simulink model "swing_equation_model_without_damping"  (R2014a)
settings: Solver=ode23t  StartTime=0.0  StopTime=3  RelTol=1e-3
settings Model: Creator=Divya M  LastModifiedBy=Divya M

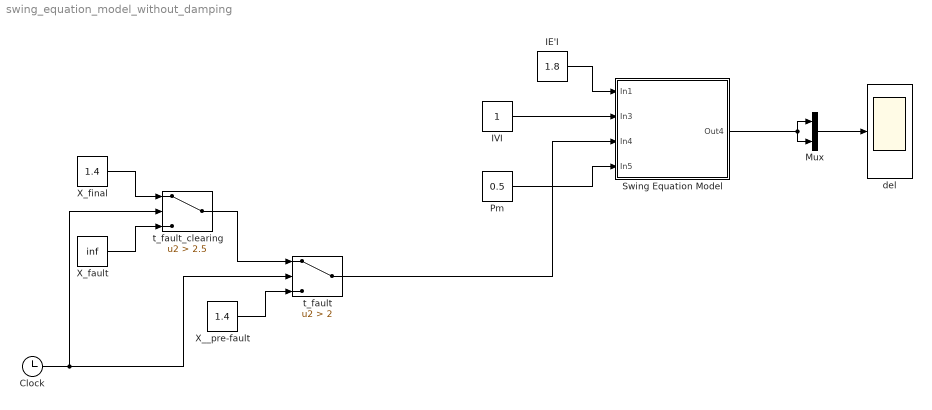
== system swing_equation_model_without_damping ==
  Clock : Clock
  IE'I : Constant  Value=1.8
  IVI : Constant
  Mux : Mux  Inputs=2
  Pm : Constant  Value=0.5
  Swing Equation Model : Subsystem
  X__pre-fault : Constant  Value=1.4
  X_fault : Constant  Value=inf
  X_final : Constant  Value=1.4
  del : Scope
      settings: TimeRange=50  YMin=-25  YMax=3120  SaveName=ScopeData2
  t_fault : Switch  Criteria=u2 > Threshold  Threshold=2
  t_fault_clearing : Switch  Criteria=u2 > Threshold  Threshold=2.5
  wires:
  IE'I/1 -> Swing Equation Model/1(In1)
  IVI/1 -> Swing Equation Model/2(In3)
  Pm/1 -> Swing Equation Model/4(In5)
  X_final/1 -> t_fault_clearing/1
  X_fault/1 -> t_fault_clearing/3
  t_fault_clearing/1 -> t_fault/1
  Clock/1 -> t_fault_clearing/2, t_fault/2
  X__pre-fault/1 -> t_fault/3
  t_fault/1 -> Swing Equation Model/3(In4)
  Swing Equation Model/1(Out4) -> Mux/2, Mux/1
  Mux/1 -> del/1

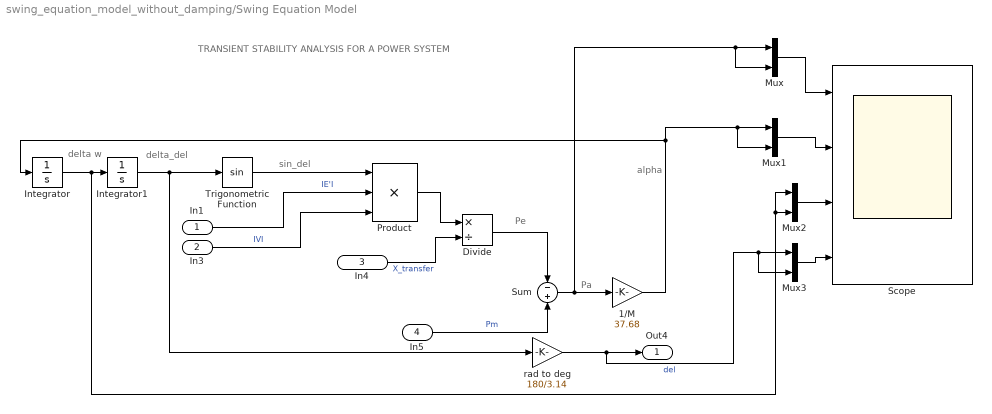
== system swing_equation_model_without_damping/Swing Equation Model ==
  note: Pa
  note: alpha
  note: Pe
  note: sin_del
  note: delta_del
  note: delta w
  note: TRANSIENT STABILITY ANALYSIS FOR A POWER SYSTEM
  In1 : Inport
  In3 : Inport  Port=2
  In4 : Inport  Port=3
  In5 : Inport  Port=4
  1/M : Gain  Gain=37.68
  Divide : Product  Inputs=*/
  Integrator : Integrator
  Integrator1 : Integrator  InitialCondition=(22.8856*pi)/180
  Mux{,1..3} (4 alike) : Mux  Inputs=2
  Product : Product  Inputs=3
  Scope : Scope  NumInputPorts=4
      settings: YMin=-5~-5~-5~-5  YMax=5~5~5~5
  Sum : Sum  Inputs=-+
  Trigonometric Function : Trigonometry
  rad to deg : Gain  Gain=180/3.14
  Out4 : Outport
  wires:
  Trigonometric Function/1 -> Product/1
  Integrator1/1 -> Trigonometric Function/1, rad to deg/1
  In4/1 -> Divide/2  "X_transfer"
  Divide/1 -> Sum/1
  Product/1 -> Divide/1
  Integrator/1 -> Mux2/2, Mux2/1, Integrator1/1
  Sum/1 -> Mux/2, Mux/1, 1/M/1
  1/M/1 -> Mux1/2, Mux1/1, Integrator/1
  In3/1 -> Product/3  "IVI"
  In1/1 -> Product/2  "IE'I"
  rad to deg/1 -> Mux3/2, Mux3/1, Out4/1  "del"
  In5/1 -> Sum/2  "Pm"
  Mux3/1 -> Scope/4
  Mux2/1 -> Scope/3
  Mux1/1 -> Scope/2
  Mux/1 -> Scope/1
